simulink model "chap05"  (R2021a)
settings: Solver=FixedStepDiscrete  StartTime=0.0  StopTime=inf  FixedStep=0.001  RelTol=1e-3
undefined symbols (not defined in the file): DiscIntNeverNeededParam, Header, Pose, X, Y, Z
libraries: robotlib x31
(part 7 of 9)

== system chap05/Subsystem16/Subsystem6/Subsystem3 ==
  utx : Inport
  vx : Inport  Port=2
  vy : Inport  Port=3
  vz : Inport  Port=4
  uty : Inport  Port=5
  ux : Inport  Port=6
  uy : Inport  Port=7
  uz : Inport  Port=8
  utz : Inport  Port=9
  switch : Inport  Port=10
  Add3 : Sum  Inputs=-+
  Add4 : Sum  Inputs=-+
  Add5 : Sum  Inputs=-+
  Demux : Demux  Outputs=3
  Demux1 : Demux  Outputs=3
  Discrete-Time Integrator1 : DiscreteIntegrator  SampleTime=-1  ICPrevOutput=DiscIntNeverNeededParam  ICPrevScaledInput=DiscIntNeverNeededParam
  Discrete-Time Integrator2 : DiscreteIntegrator  SampleTime=-1  ICPrevOutput=DiscIntNeverNeededParam  ICPrevScaledInput=DiscIntNeverNeededParam
  Discrete-Time Integrator8 : DiscreteIntegrator  SampleTime=-1  ICPrevOutput=DiscIntNeverNeededParam  ICPrevScaledInput=DiscIntNeverNeededParam
  MATLAB Function : MATLAB Function  TreatAsAtomicUnit=on
  MATLAB Function1 : MATLAB Function  TreatAsAtomicUnit=on
  MATLAB Function2 : MATLAB Function  TreatAsAtomicUnit=on
  Mux : Mux  Inputs=3
  Mux1 : Mux  Inputs=3
  Subsystem : Subsystem
  Subsystem1 : Subsystem
  Subsystem2 : Subsystem
      settings: PortSchema="{\"entries\":[{\"content\":{\"sides\":[{\"content\":{\"connectorIds\":[\"In1\"]},\"type\":\"ConnectorPlacement.EquallySpacedRectSide\",\"uuid\":\"fc08b57d-5108-4bb3-894e-d1527c9ee9b9\"},{\"content\":{\"connectorIds\":[\"Out1\",\"Out2\",\"Out3\",\"Out4\"],\"side\":\"RIGHT\"},\"type\":\"ConnectorPlacement.EquallySpacedRectSide\",\"uuid\":\"5f28f464-9d6d-4ee7-848e-113b4b51ead6\"},{\"content\":{\"connectorIds\":[],\"side\":\"TOP\"},\"type\":\"ConnectorPlacement.EquallySpacedRectSide\",\"uuid\":\"5cca314e-822b-43eb-ac4d-78622e8ed582\"},{\"content\":{\"connectorIds\":[\"In2\"],\"side\":\"BOTTOM\"},\"type\":\"ConnectorPlacement.EquallySpacedRectSide\",\"uuid\":\"aa07b2d0-4f6e-4d8e-96de-14c35ee3da88\"}]},\"type\":\"ConnectorPlacement.EquallySpacedConnector\",\"uuid\":\"246d6f2c-2f9e-403c-b810-eff9b0fc0735\"}],\"packageUris\":[\"http://schema.mathworks.com/mf0/Connector/R2020b\"],\"version\":\"1.0\"}"
  Subsystem3 : Subsystem
  Subtract1 : Sum  Inputs=++++
  Subtract2 : Sum  Inputs=+-
  Subtract3 : Sum  Inputs=+-
  Subtract4 : Sum  Inputs=+-
  Switch1 : Switch  Criteria=u2 > Threshold  Threshold=1
  Switch2 : Switch  Criteria=u2 > Threshold  Threshold=1
  Switch3 : Switch  Criteria=u2 > Threshold  Threshold=1
  udtx : Outport
  udty : Outport  Port=2
  udtz : Outport  Port=3
  wires:
  Subsystem3/1(Out1) -> Subtract1/2
  Subsystem2/2(k2) -> Subsystem3/2(k2)
  Subsystem1/1(Out1) -> Subtract1/1
  Subsystem2/1(k1) -> Subsystem1/2(k1)
  Subtract4/1 -> MATLAB Function2/1(u)
  Subtract3/1 -> MATLAB Function1/1(u)
  Subtract2/1 -> MATLAB Function/1(u)
  Demux/3 -> Discrete-Time Integrator8/1
  Demux/1 -> Discrete-Time Integrator2/1
  Demux/2 -> Discrete-Time Integrator1/1
  Discrete-Time Integrator2/1 -> Subtract2/1
  Discrete-Time Integrator1/1 -> Subtract3/1
  Discrete-Time Integrator8/1 -> Subtract4/1
  Mux1/1 -> Subtract1/4
  ux/1 -> Mux1/1
  uy/1 -> Mux1/2
  uz/1 -> Mux1/3
  vx/1 -> Subtract2/2
  Subsystem2/4(k4) -> Subsystem/3(k4)
  Subsystem/1(z2) -> Demux1/1, Subtract1/3  "od6"
  Subsystem2/3(k3) -> Subsystem/2(k3)
  Subtract1/1 -> Demux/1
  Mux/1 -> Subsystem1/1(e1), Subsystem3/1(e1), Subsystem2/1(e1), Subsystem/1(e1)
  utx/1 -> Switch1/3, Add3/2
  uty/1 -> Switch2/3, Add5/2
  utz/1 -> Switch3/3, Add4/2
  vy/1 -> Subtract3/2
  vz/1 -> Subtract4/2
  MATLAB Function/1(y) -> Mux/1
  MATLAB Function1/1(y) -> Mux/2
  MATLAB Function2/1(y) -> Mux/3
  switch/1 -> [switch], Switch3/2, Switch1/2, Switch2/2
  [switch] -> Subsystem2/2(switch)
  Add3/1 -> Switch1/1
  Add5/1 -> Switch2/1
  Add4/1 -> Switch3/1
  Switch1/1 -> udtx/1
  Switch2/1 -> udty/1
  Switch3/1 -> udtz/1
  Demux1/1 -> Add3/1
  Demux1/2 -> Add5/1
  Demux1/3 -> Add4/1

== system chap05/Subsystem16/Subsystem6/Subsystem4 ==
  vx6 : Inport
  vx0 : Inport  Port=2
  utx : Inport  Port=3
  gain : Inport  Port=4
  switch : Inport  Port=5
  Add1 : Sum  Inputs=--+
  Constant1 : Constant  Value=0.08
  Constant2 : Constant  Value=10
  Product : Product
  Product1 : Product
  Product2 : Product
  Subsystem : Subsystem
  Subtract : Sum  Inputs=+--
  Switch1 : Switch  Criteria=u2 > Threshold  Threshold=1
  Tanh : Trigonometry  Operator=tanh
  ux : Outport
  Sx : Outport  Port=2
  wires:
  Add1/1 -> Switch1/1
  utx/1 -> [A], Subsystem/2(zt3)
  Subsystem/1(Out1) -> Subtract/3
  Product/1 -> Add1/2
  vx6/1 -> Subtract/1
  Product2/1 -> Tanh/1
  Tanh/1 -> Product/1
  gain/1 -> Product/2
  [A] -> Add1/3
  Constant2/1 -> Product2/2
  Product1/1 -> Add1/1
  Subtract/1 -> Sx/1, Product1/2, Product2/1
  vx0/1 -> Subtract/2
  switch/1 -> [switch], Subsystem/1(switch)
  [A] -> Switch1/3
  [switch] -> Switch1/2
  Switch1/1 -> ux/1
  Constant1/1 -> Product1/1

== system chap05/Subsystem16/Subsystem6/Subsystem5 ==
  vy6 : Inport
  vy0 : Inport  Port=2
  uty : Inport  Port=3
  gain : Inport  Port=4
  switch : Inport  Port=5
  Add1 : Sum  Inputs=--+
  Constant1 : Constant  Value=0.08
  Constant2 : Constant  Value=10
  Product : Product
  Product1 : Product
  Product2 : Product
  Subsystem : Subsystem
  Subtract : Sum  Inputs=+--
  Switch1 : Switch  Criteria=u2 > Threshold  Threshold=1
  Tanh : Trigonometry  Operator=tanh
  uy : Outport
  Sz : Outport  Port=2
  wires:
  Switch1/1 -> uy/1
  [switch] -> Switch1/2
  [A] -> Switch1/3
  switch/1 -> Subsystem/1(switch), [switch]
  vy0/1 -> Subtract/2
  Subtract/1 -> Product2/1, Product1/2, Sz/1
  Constant1/1 -> Product1/1
  Product1/1 -> Add1/1
  Constant2/1 -> Product2/2
  [A] -> Add1/3
  gain/1 -> Product/2
  Tanh/1 -> Product/1
  Product2/1 -> Tanh/1
  vy6/1 -> Subtract/1
  Product/1 -> Add1/2
  Subsystem/1(Out1) -> Subtract/3
  uty/1 -> Subsystem/2(zt3), [A]
  Add1/1 -> Switch1/1

== system chap05/Subsystem16/Subsystem6/Subsystem6 ==
  xx6 : Inport
  xx0 : Inport  Port=2
  xx1 : Inport  Port=3
  xx2 : Inport  Port=4
  vx6 : Inport  Port=5
  vx0 : Inport  Port=6
  vx1 : Inport  Port=7
  vx2 : Inport  Port=8
  Add : Sum
  Add1 : Sum  Inputs=-+
  Add10 : Sum  Inputs=-+
  Add2 : Sum  Inputs=+-
  Add4 : Sum  Inputs=-+
  Add5 : Sum  Inputs=+++
  Add6 : Sum  Inputs=+-
  Add8 : Sum  Inputs=+++
  Add9 : Sum  Inputs=+-
  Constant : Constant  Value=0.75
  Constant1 : Constant  Value=0.85
  Constant3 : Constant  Value=1.2
  Constant{4..5,7..8} (4 alike) : Constant  Value=1.5
  Constant6 : Constant  Value=1.2
  Gain : Gain  Gain=-1
  Product{1,3..9} (8 alike) : Product
  utx : Outport
  wires:
  Product9/1 -> Add8/2
  Product8/1 -> Add8/1
  Add9/1 -> Product9/1
  Constant6/1 -> Product9/2
  Add10/1 -> Product8/2
  Constant5/1 -> Product8/1
  Add8/1 -> Product1/2
  Product4/1 -> Add5/2
  Product5/1 -> Add5/3
  Constant4/1 -> Product4/1
  Add4/1 -> Product4/2
  xx6/1 -> Add1/2, Add2/1, Add4/2
  Constant3/1 -> Product5/2
  Product6/1 -> Add/1
  Constant/1 -> Product6/1
  Constant1/1 -> Product1/1
  Product1/1 -> Add/2
  Add2/1 -> Product5/1
  Add5/1 -> Product6/2
  xx2/1 -> Add4/1
  xx1/1 -> Add2/2
  vx1/1 -> Add9/2
  vx2/1 -> Add10/1
  vx6/1 -> Add6/1, Add9/1, Add10/2
  xx0/1 -> Add1/1
  Constant7/1 -> Product3/1
  Add1/1 -> Product3/2
  Product3/1 -> Add5/1
  vx0/1 -> Add6/2
  Constant8/1 -> Product7/2
  Add6/1 -> Product7/1
  Product7/1 -> Add8/3
  Gain/1 -> utx/1
  Add/1 -> Gain/1

== system chap05/Subsystem16/Subsystem6/Subsystem7 ==
  vz6 : Inport
  vz0 : Inport  Port=2
  utz : Inport  Port=3
  gain : Inport  Port=4
  switch : Inport  Port=5
  Add1 : Sum  Inputs=--+
  Constant1 : Constant  Value=0.08
  Constant2 : Constant  Value=10
  Product : Product
  Product1 : Product
  Product2 : Product
  Subsystem : Subsystem
  Subtract : Sum  Inputs=+--
  Switch1 : Switch  Criteria=u2 > Threshold  Threshold=1
  Tanh : Trigonometry  Operator=tanh
  uz : Outport
  Sz : Outport  Port=2
  wires:
  Add1/1 -> Switch1/1
  utz/1 -> [A], Subsystem/2(zt3)
  Subsystem/1(Out1) -> Subtract/3
  Product/1 -> Add1/2
  vz6/1 -> Subtract/1
  Product2/1 -> Tanh/1
  Tanh/1 -> Product/1
  gain/1 -> Product/2
  [A] -> Add1/3
  Constant2/1 -> Product2/2
  Product1/1 -> Add1/1
  Constant1/1 -> Product1/1
  Subtract/1 -> Sz/1, Product1/2, Product2/1
  vz0/1 -> Subtract/2
  switch/1 -> [switch], Subsystem/1(switch)
  [A] -> Switch1/3
  [switch] -> Switch1/2
  Switch1/1 -> uz/1

== system chap05/Subsystem16/Subsystem6/Subsystem8 ==
  Sx : Inport
  Sy : Inport  Port=2
  Sz : Inport  Port=3
  vx : Inport  Port=4
  vy : Inport  Port=5
  vz : Inport  Port=6
  switch : Inport  Port=7
  Constant{,1..3} (4 alike) : Constant  Value=0.1
  Discrete-Time Integrator1 : DiscreteIntegrator  gainval=1  InitialCondition=0.05  SampleTime=-1  ICPrevOutput=DiscIntNeverNeededParam  ICPrevScaledInput=DiscIntNeverNeededParam
  Discrete-Time Integrator2 : DiscreteIntegrator  gainval=1  InitialCondition=0.025  SampleTime=-1  ICPrevOutput=DiscIntNeverNeededParam  ICPrevScaledInput=DiscIntNeverNeededParam
  Discrete-Time Integrator3 : DiscreteIntegrator  gainval=1  InitialCondition=0.01  SampleTime=-1  ICPrevOutput=DiscIntNeverNeededParam  ICPrevScaledInput=DiscIntNeverNeededParam
  MATLAB Function : MATLAB Function  TreatAsAtomicUnit=on
  MATLAB Function1 : MATLAB Function  TreatAsAtomicUnit=on
  Mux1 : Mux  Inputs=3
  Mux3 : Mux  Inputs=3
  Product{1..4,6..8} (7 alike) : Product
  Square : Math  Operator=square  SaturateOnIntegerOverflow=on
  Square1 : Math  Operator=square  SaturateOnIntegerOverflow=on
  Subsystem : Subsystem
      settings: PortSchema="{\"entries\":[{\"content\":{\"sides\":[{\"content\":{\"connectorIds\":[\"In1\"]},\"type\":\"ConnectorPlacement.EquallySpacedRectSide\",\"uuid\":\"50b1559e-7173-4ba8-93e6-314f6d9df527\"},{\"content\":{\"connectorIds\":[\"Out1\"],\"side\":\"RIGHT\"},\"type\":\"ConnectorPlacement.EquallySpacedRectSide\",\"uuid\":\"be527bac-0bcc-4faf-a185-0382edae0189\"},{\"content\":{\"connectorIds\":[\"In2\"],\"side\":\"TOP\"},\"type\":\"ConnectorPlacement.EquallySpacedRectSide\",\"uuid\":\"4c8ef68d-7cf5-4d15-9758-89dbc1169805\"}]},\"type\":\"ConnectorPlacement.EquallySpacedConnector\",\"uuid\":\"3c2ee67b-c3c9-431a-8107-6d5cd22b236e\"}],\"packageUris\":[\"http://schema.mathworks.com/mf0/Connector/R2020b\"],\"version\":\"1.0\"}"
  Subsystem1 : Subsystem
      settings: PortSchema="{\"entries\":[{\"content\":{\"sides\":[{\"content\":{\"connectorIds\":[\"In1\"]},\"type\":\"ConnectorPlacement.EquallySpacedRectSide\",\"uuid\":\"50b1559e-7173-4ba8-93e6-314f6d9df527\"},{\"content\":{\"connectorIds\":[\"Out1\"],\"side\":\"RIGHT\"},\"type\":\"ConnectorPlacement.EquallySpacedRectSide\",\"uuid\":\"be527bac-0bcc-4faf-a185-0382edae0189\"},{\"content\":{\"connectorIds\":[\"In2\"],\"side\":\"TOP\"},\"type\":\"ConnectorPlacement.EquallySpacedRectSide\",\"uuid\":\"4c8ef68d-7cf5-4d15-9758-89dbc1169805\"}]},\"type\":\"ConnectorPlacement.EquallySpacedConnector\",\"uuid\":\"3c2ee67b-c3c9-431a-8107-6d5cd22b236e\"}],\"packageUris\":[\"http://schema.mathworks.com/mf0/Connector/R2020b\"],\"version\":\"1.0\"}"
  Subsystem2 : Subsystem
      settings: PortSchema="{\"entries\":[{\"content\":{\"sides\":[{\"content\":{\"connectorIds\":[\"In1\"]},\"type\":\"ConnectorPlacement.EquallySpacedRectSide\",\"uuid\":\"50b1559e-7173-4ba8-93e6-314f6d9df527\"},{\"content\":{\"connectorIds\":[\"Out1\"],\"side\":\"RIGHT\"},\"type\":\"ConnectorPlacement.EquallySpacedRectSide\",\"uuid\":\"be527bac-0bcc-4faf-a185-0382edae0189\"},{\"content\":{\"connectorIds\":[\"In2\"],\"side\":\"TOP\"},\"type\":\"ConnectorPlacement.EquallySpacedRectSide\",\"uuid\":\"4c8ef68d-7cf5-4d15-9758-89dbc1169805\"}]},\"type\":\"ConnectorPlacement.EquallySpacedConnector\",\"uuid\":\"3c2ee67b-c3c9-431a-8107-6d5cd22b236e\"}],\"packageUris\":[\"http://schema.mathworks.com/mf0/Connector/R2020b\"],\"version\":\"1.0\"}"
  Subtract1 : Sum  Inputs=++++
  Subtract2 : Sum  Inputs=+-
  Subtract3 : Sum  Inputs=+-
  Subtract4 : Sum  Inputs=+-
  " gain" : Outport
  wires:
  [switch] -> Subsystem2/2(switch)
  [switch] -> Subsystem1/2(switch)
  [switch] -> Subsystem/2(switch)
  switch/1 -> [switch]
  Subsystem1/1(Out1) -> Discrete-Time Integrator2/1
  Subsystem2/1(Out1) -> Discrete-Time Integrator3/1
  Subsystem/1(Out1) -> Discrete-Time Integrator1/1
  [norm_V] -> Product8/2
  Square1/1 -> Product4/1
  [norm_V] -> Square1/1
  [norm_V] -> Product1/1
  [norm_V] -> Square/1
  [norm_S] -> Product3/1
  [norm_S] -> Product8/1
  [norm_S] -> Subtract2/1
  MATLAB Function/1(y) -> [norm_S]
  vy/1 -> Mux1/2
  vz/1 -> Mux1/3
  vx/1 -> Mux1/1
  Sz/1 -> Mux3/3
  Sy/1 -> Mux3/2
  Sx/1 -> Mux3/1
  Constant3/1 -> Product7/1
  Constant2/1 -> Product6/1
  Constant1/1 -> Subtract1/4
  Product4/1 -> Subtract1/3
  MATLAB Function1/1(y) -> [norm_V]
  Constant/1 -> Product2/1
  Mux1/1 -> MATLAB Function1/1(u)
  Square/1 -> Product3/2
  Mux3/1 -> MATLAB Function/1(u)
  Discrete-Time Integrator3/1 -> Product2/2, Product4/2  "K2"
  Product2/1 -> Subtract4/2
  Product3/1 -> Subtract4/1
  Subtract4/1 -> Subsystem2/1(In1)
  Subtract3/1 -> Subsystem1/1(In1)
  Product8/1 -> Subtract3/1
  Product7/1 -> Subtract3/2
  Discrete-Time Integrator2/1 -> Product1/2, Product7/2  "K1"
  Product6/1 -> Subtract2/2
  Discrete-Time Integrator1/1 -> Subtract1/1, Product6/2  "K0"
  Subtract2/1 -> Subsystem/1(In1)
  Product1/1 -> Subtract1/2
  Subtract1/1 -> " gain"/1

== system chap05/Subsystem16/Subsystem8/L+B ==
  Add : Sum
  Constant1 : Constant  Value=|
      | [2.5 0 0 0 0 0
      |      0 2.8 0 0 0 0
      |      0 0 2.8 0 0 0
      |      0 0 0 2.5 0 0
      |      0 0 0 0 2.7 0
      |      0 0 0 0 0 2.7]
  Constant2 : Constant  Value=|
      | [0.0 0.8 0.5 0.0 0.0 1.2
      |      0.8 0.0 0.0 0.5 0.0 1.5
      |      0.5 0.0 0.0 0.8 1.5 0.0
      |      0.0 0.5 0.8 0.0 1.2 0.0
      |      0.0 0.0 1.5 1.2 0.0 0.0
      |      1.2 1.5 0.0 0.0 0.0 0.0]
  Constant3 : Constant  Value=|
      | [0.0 0.0 0.0 0.0 0.0 0.0
      |      0.0 0.0 0.0 0.0 0.0 0.0
      |      0.0 0.0 0.0 0.0 0.0 0.0
      |      0.0 0.0 0.0 0.0 0.0 0.0
      |      0.0 0.0 0.0 0.0 1.5 0.0
      |      0.0 0.0 0.0 0.0 0.0 1.5]
  Subtract : Sum  Inputs=+-
  u : Outport
  wires:
  Constant2/1 -> Subtract/2
  Constant1/1 -> Subtract/1
  Subtract/1 -> Add/1
  Add/1 -> u/1
  Constant3/1 -> Add/2

== system chap05/Subsystem16/Subsystem8/Subsystem1 ==
  xy4 : Inport
  xy2 : Inport  Port=2
  xy3 : Inport  Port=3
  xy5 : Inport  Port=4
  vy4 : Inport  Port=5
  vy2 : Inport  Port=6
  vy3 : Inport  Port=7
  vy5 : Inport  Port=8
  Add : Sum
  Add{1,4,6,8} (4 alike) : Sum  Inputs=-+
  Add2 : Sum  Inputs=+-
  Add5 : Sum  Inputs=+++
  Add7 : Sum  Inputs=+-
  Add9 : Sum  Inputs=+++
  Constant : Constant  Value=0.75
  Constant1 : Constant  Value=0.85
  Constant2 : Constant  Value=0.8
  Constant3 : Constant  Value=0.8
  Constant4 : Constant  Value=0.5
  Constant5 : Constant  Value=1.2
  Constant6 : Constant  Value=0.5
  Constant7 : Constant  Value=1.2
  Product{1,3..9} (8 alike) : Product
  p4y : Outport
  wires:
  Product8/1 -> Add9/2
  Product9/1 -> Add9/3
  Constant2/1 -> Product8/1
  Add8/1 -> Product8/2
  vy4/1 -> Add6/2, Add8/2, Add7/1
  Constant6/1 -> Product9/2
  Add7/1 -> Product9/1
  vy3/1 -> Add8/1
  vy2/1 -> Add7/2
  vy5/1 -> Add6/1
  Constant7/1 -> Product7/1
  Add6/1 -> Product7/2
  Product7/1 -> Add9/1
  Product3/1 -> Add5/1
  Add1/1 -> Product3/2
  Constant5/1 -> Product3/1
  xy5/1 -> Add1/1
  xy2/1 -> Add2/2
  xy3/1 -> Add4/1
  Add/1 -> p4y/1
  Add5/1 -> Product6/2
  Add2/1 -> Product5/1
  Product1/1 -> Add/2
  Constant1/1 -> Product1/1
  Constant/1 -> Product6/1
  Product6/1 -> Add/1
  Constant4/1 -> Product5/2
  xy4/1 -> Add2/1, Add4/2, Add1/2
  Add4/1 -> Product4/2
  Constant3/1 -> Product4/1
  Product5/1 -> Add5/3
  Product4/1 -> Add5/2
  Add9/1 -> Product1/2

== system chap05/Subsystem16/Subsystem8/Subsystem2 ==
  xz4 : Inport
  xx2 : Inport  Port=2
  xz3 : Inport  Port=3
  xz5 : Inport  Port=4
  vz4 : Inport  Port=5
  vz2 : Inport  Port=6
  vz3 : Inport  Port=7
  vz5 : Inport  Port=8
  Add : Sum
  Add{1,4,6,8} (4 alike) : Sum  Inputs=-+
  Add2 : Sum  Inputs=+-
  Add5 : Sum  Inputs=+++
  Add7 : Sum  Inputs=+-
  Add9 : Sum  Inputs=+++
  Constant : Constant  Value=0.75
  Constant1 : Constant  Value=0.85
  Constant2 : Constant  Value=0.8
  Constant3 : Constant  Value=0.8
  Constant4 : Constant  Value=0.5
  Constant5 : Constant  Value=1.2
  Constant6 : Constant  Value=0.5
  Constant7 : Constant  Value=1.2
  Product{1,3..9} (8 alike) : Product
  p4z : Outport
  wires:
  Add9/1 -> Product1/2
  Product4/1 -> Add5/2
  Product5/1 -> Add5/3
  Constant3/1 -> Product4/1
  Add4/1 -> Product4/2
  xz4/1 -> Add1/2, Add4/2, Add2/1
  Constant4/1 -> Product5/2
  Product6/1 -> Add/1
  Constant/1 -> Product6/1
  Constant1/1 -> Product1/1
  Product1/1 -> Add/2
  Add2/1 -> Product5/1
  Add5/1 -> Product6/2
  Add/1 -> p4z/1
  xz3/1 -> Add4/1
  xx2/1 -> Add2/2
  xz5/1 -> Add1/1
  Constant5/1 -> Product3/1
  Add1/1 -> Product3/2
  Product3/1 -> Add5/1
  Product7/1 -> Add9/1
  Add6/1 -> Product7/2
  Constant7/1 -> Product7/1
  vz5/1 -> Add6/1
  vz2/1 -> Add7/2
  vz3/1 -> Add8/1
  Add7/1 -> Product9/1
  Constant6/1 -> Product9/2
  vz4/1 -> Add7/1, Add8/2, Add6/2
  Add8/1 -> Product8/2
  Constant2/1 -> Product8/1
  Product9/1 -> Add9/3
  Product8/1 -> Add9/2

== system chap05/Subsystem16/Subsystem8/Subsystem3 ==
  xyk : Inport
  xy : Inport  Port=2
  vyk : Inport  Port=3
  vy : Inport  Port=4
  Add : Sum
  Add4 : Sum  Inputs=-+
  Add8 : Sum  Inputs=-+
  Constant : Constant  Value=0.75
  Constant1 : Constant  Value=0.85
  Product1 : Product
  Product6 : Product
  ey : Outport
  wires:
  vyk/1 -> Add8/2
  vy/1 -> Add8/1
  xy/1 -> Add4/1
  Add/1 -> ey/1
  Add4/1 -> Product6/2
  Product1/1 -> Add/2
  Constant1/1 -> Product1/1
  Constant/1 -> Product6/1
  Product6/1 -> Add/1
  xyk/1 -> Add4/2
  Add8/1 -> Product1/2

== system chap05/Subsystem16/Subsystem8/Subsystem4 ==
  xzk : Inport
  xz : Inport  Port=2
  vzk : Inport  Port=3
  vz : Inport  Port=4
  Add : Sum
  Add4 : Sum  Inputs=-+
  Add8 : Sum  Inputs=-+
  Constant : Constant  Value=0.75
  Constant1 : Constant  Value=0.85
  Product1 : Product
  Product6 : Product
  ez : Outport
  wires:
  Add8/1 -> Product1/2
  xzk/1 -> Add4/2
  Product6/1 -> Add/1
  Constant/1 -> Product6/1
  Constant1/1 -> Product1/1
  Product1/1 -> Add/2
  Add4/1 -> Product6/2
  Add/1 -> ez/1
  xz/1 -> Add4/1
  vz/1 -> Add8/1
  vzk/1 -> Add8/2

== system chap05/Subsystem16/Subsystem8/Subsystem5 ==
  xxk : Inport
  xx : Inport  Port=2
  vxk : Inport  Port=3
  vx : Inport  Port=4
  Add : Sum
  Add4 : Sum  Inputs=-+
  Add8 : Sum  Inputs=-+
  Constant : Constant  Value=0.75
  Constant1 : Constant  Value=0.85
  Product1 : Product
  Product6 : Product
  ex : Outport
  wires:
  Add8/1 -> Product1/2
  xxk/1 -> Add4/2
  Product6/1 -> Add/1
  Constant/1 -> Product6/1
  Constant1/1 -> Product1/1
  Product1/1 -> Add/2
  Add4/1 -> Product6/2
  Add/1 -> ex/1
  xx/1 -> Add4/1
  vx/1 -> Add8/1
  vxk/1 -> Add8/2

== system chap05/Subsystem16/Subsystem8/Subsystem6 ==
  xx4 : Inport
  xx2 : Inport  Port=2
  xx3 : Inport  Port=3
  xx5 : Inport  Port=4
  vx4 : Inport  Port=5
  vx2 : Inport  Port=6
  vx3 : Inport  Port=7
  vx5 : Inport  Port=8
  Add : Sum
  Add{1,4,6,8} (4 alike) : Sum  Inputs=-+
  Add2 : Sum  Inputs=+-
  Add5 : Sum  Inputs=+++
  Add7 : Sum  Inputs=+-
  Add9 : Sum  Inputs=+++
  Constant : Constant  Value=0.75
  Constant1 : Constant  Value=0.85
  Constant2 : Constant  Value=0.8
  Constant3 : Constant  Value=0.8
  Constant4 : Constant  Value=0.5
  Constant5 : Constant  Value=1.2
  Constant6 : Constant  Value=0.5
  Constant7 : Constant  Value=1.2
  Product{1,3..9} (8 alike) : Product
  p4x : Outport
  wires:
  Add9/1 -> Product1/2
  Product4/1 -> Add5/2
  Product5/1 -> Add5/3
  Constant3/1 -> Product4/1
  Add4/1 -> Product4/2
  xx4/1 -> Add1/2, Add4/2, Add2/1
  Constant4/1 -> Product5/2
  Product6/1 -> Add/1
  Constant/1 -> Product6/1
  Constant1/1 -> Product1/1
  Product1/1 -> Add/2
  Add2/1 -> Product5/1
  Add5/1 -> Product6/2
  Add/1 -> p4x/1
  xx3/1 -> Add4/1
  xx2/1 -> Add2/2
  xx5/1 -> Add1/1
  Constant5/1 -> Product3/1
  Add1/1 -> Product3/2
  Product3/1 -> Add5/1
  Product7/1 -> Add9/1
  Add6/1 -> Product7/2
  Constant7/1 -> Product7/1
  vx5/1 -> Add6/1
  vx2/1 -> Add7/2
  vx3/1 -> Add8/1
  Add7/1 -> Product9/1
  Constant6/1 -> Product9/2
  vx4/1 -> Add7/1, Add8/2, Add6/2
  Add8/1 -> Product8/2
  Constant2/1 -> Product8/1
  Product9/1 -> Add9/3
  Product8/1 -> Add9/2

== system chap05/Subsystem16/Subsystem/Subsystem11/Subsystem ==
  switch : Inport
  zt3 : Inport  Port=2
  Constant4 : Constant  Value=0
  Discrete-Time Integrator : DiscreteIntegrator  SampleTime=-1  UpperSaturationLimit=100  LowerSaturationLimit=-100  ICPrevOutput=DiscIntNeverNeededParam  ICPrevScaledInput=DiscIntNeverNeededParam
  Logical Operator : Logic  AllPortsSameDT=off  OutDataTypeStr=boolean
  MATLAB Function : MATLAB Function  TreatAsAtomicUnit=on
  Relational Operator : RelationalOperator  Operator===  OutDataTypeStr=boolean  RndMeth=Simplest
  Saturation1 : Saturate  UpperLimit=0.25  LowerLimit=-0.25
  Sign : Signum
  Sign1 : Signum
  Subsystem : Subsystem
      settings: PortSchema="{\"entries\":[{\"content\":{\"sides\":[{\"content\":{\"connectorIds\":[\"In1\"]},\"type\":\"ConnectorPlacement.EquallySpacedRectSide\",\"uuid\":\"50b1559e-7173-4ba8-93e6-314f6d9df527\"},{\"content\":{\"connectorIds\":[\"Out1\"],\"side\":\"RIGHT\"},\"type\":\"ConnectorPlacement.EquallySpacedRectSide\",\"uuid\":\"be527bac-0bcc-4faf-a185-0382edae0189\"},{\"content\":{\"connectorIds\":[\"In2\"],\"side\":\"TOP\"},\"type\":\"ConnectorPlacement.EquallySpacedRectSide\",\"uuid\":\"4c8ef68d-7cf5-4d15-9758-89dbc1169805\"}]},\"type\":\"ConnectorPlacement.EquallySpacedConnector\",\"uuid\":\"3c2ee67b-c3c9-431a-8107-6d5cd22b236e\"}],\"packageUris\":[\"http://schema.mathworks.com/mf0/Connector/R2020b\"],\"version\":\"1.0\"}"
  Switch : Switch  Criteria=u2 > Threshold
  Out1 : Outport
  wires:
  MATLAB Function/1(y) -> Logical Operator/1
  Relational Operator/1 -> Logical Operator/2
  Constant4/1 -> Switch/1
  Sign1/1 -> Relational Operator/1
  Subsystem/1(Out1) -> Sign1/1, Switch/3
  Saturation1/1 -> Out1/1, MATLAB Function/2(u2)
  Discrete-Time Integrator/1 -> Saturation1/1, MATLAB Function/1(u1), Sign/1
  Sign/1 -> Relational Operator/2
  Logical Operator/1 -> Switch/2
  Switch/1 -> Discrete-Time Integrator/1
  zt3/1 -> Subsystem/1(zt3)
  switch/1 -> Subsystem/2(switch)

== system chap05/Subsystem16/Subsystem/Subsystem3/Subsystem ==
  e1 : Inport
  k3 : Inport  Port=2
  k4 : Inport  Port=3
  Add : Sum
  Constant3 : Constant  Value=-1
  Constant4 : Constant  Value=-1
  Discrete-Time Integrator1 : DiscreteIntegrator  SampleTime=-1  ICPrevOutput=DiscIntNeverNeededParam  ICPrevScaledInput=DiscIntNeverNeededParam
  Divide : Product  Inputs=*/
  MATLAB Function : MATLAB Function  TreatAsAtomicUnit=on
  Product3 : Product  Inputs=3
  Product5 : Product  Inputs=3
  z2 : Outport
  wires:
  Constant4/1 -> Product5/1
  Product5/1 -> Add/2
  Discrete-Time Integrator1/1 -> z2/1
  k3/1 -> Product3/3
  k4/1 -> Product5/3
  Divide/1 -> Add/1
  Add/1 -> Discrete-Time Integrator1/1
  Constant3/1 -> Product3/1
  e1/1 -> Product5/2, MATLAB Function/1(u), Product3/2
  MATLAB Function/1(y) -> Divide/2
  Product3/1 -> Divide/1

== system chap05/Subsystem16/Subsystem/Subsystem3/Subsystem1 ==
  e1 : Inport
  k1 : Inport  Port=2
  Constant : Constant  Value=-1
  Divide : Product  Inputs=*/
  MATLAB Function : MATLAB Function  TreatAsAtomicUnit=on
  Product : Product  Inputs=3
  Out1 : Outport
  wires:
  e1/1 -> Product/2, MATLAB Function/1(u)
  Divide/1 -> Out1/1
  Constant/1 -> Product/1
  k1/1 -> Product/3
  MATLAB Function/1(y) -> Divide/2
  Product/1 -> Divide/1

== system chap05/Subsystem16/Subsystem/Subsystem3/Subsystem2 ==
  e1 : Inport
  switch : Inport  Port=2
  Constant1 : Constant  Value=0.1
  MATLAB Function : MATLAB Function  TreatAsAtomicUnit=on
  Product{,1..3,6} (5 alike) : Product
  Sqrt : Sqrt  SaturateOnIntegerOverflow=on
  Square : Math  Operator=square  SaturateOnIntegerOverflow=on
  Subsystem : Subsystem
      settings: PortSchema="{\"entries\":[{\"content\":{\"sides\":[{\"content\":{\"connectorIds\":[\"In1\"]},\"type\":\"ConnectorPlacement.EquallySpacedRectSide\",\"uuid\":\"12a3f2f0-a297-420d-b26a-5f62088d5514\"},{\"content\":{\"connectorIds\":[\"Out1\"],\"side\":\"RIGHT\"},\"type\":\"ConnectorPlacement.EquallySpacedRectSide\",\"uuid\":\"62e35448-e0a3-4495-a6db-77deef7aa7b4\"},{\"content\":{\"connectorIds\":[\"In2\"],\"side\":\"TOP\"},\"type\":\"ConnectorPlacement.EquallySpacedRectSide\",\"uuid\":\"3e6c604a-b26b-4ac2-9bdc-2cdec7247e53\"}]},\"type\":\"ConnectorPlacement.EquallySpacedConnector\",\"uuid\":\"6331fe4a-63c7-4003-9b0d-be968a8635fa\"}],\"packageUris\":[\"http://schema.mathworks.com/mf0/Connector/R2020b\"],\"version\":\"1.0\"}"
  Subtract2 : Sum  Inputs=+-
  c1 : Constant  Value=0.1
  c2 : Constant  Value=0.1
  c3 : Constant  Value=0.3
  c4 : Constant  Value=0.3
  k1 : Outport
  k2 : Outport  Port=2
  k3 : Outport  Port=3
  k4 : Outport  Port=4
  wires:
  c2/1 -> Product/2
  Product/1 -> k2/1
  c3/1 -> Product1/1
  Product1/1 -> k3/1
  c4/1 -> Product2/1
  Product2/1 -> k4/1
  c1/1 -> Product3/2
  Product3/1 -> k1/1
  Sqrt/1 -> Product3/1
  Square/1 -> Product2/2
  e1/1 -> MATLAB Function/1(u)
  Product6/1 -> Subtract2/2
  MATLAB Function/1(y) -> Subtract2/1
  Subtract2/1 -> Subsystem/1(In1)
  Constant1/1 -> Product6/1
  switch/1 -> Subsystem/2(switch)
  Subsystem/1(Out1) -> Product6/2, Sqrt/1, Product1/2, Square/1, Product/1

== system chap05/Subsystem16/Subsystem/Subsystem3/Subsystem3 ==
  e1 : Inport
  k2 : Inport  Port=2
  Constant2 : Constant  Value=-1
  Product2 : Product  Inputs=3
  Out1 : Outport
  wires:
  Product2/1 -> Out1/1
  e1/1 -> Product2/2
  k2/1 -> Product2/3
  Constant2/1 -> Product2/1

== system chap05/Subsystem16/Subsystem/Subsystem4/Subsystem ==
  switch : Inport
  zt3 : Inport  Port=2
  Constant4 : Constant  Value=0
  Discrete-Time Integrator : DiscreteIntegrator  SampleTime=-1  UpperSaturationLimit=100  LowerSaturationLimit=-100  ICPrevOutput=DiscIntNeverNeededParam  ICPrevScaledInput=DiscIntNeverNeededParam
  Logical Operator : Logic  AllPortsSameDT=off  OutDataTypeStr=boolean
  MATLAB Function : MATLAB Function  TreatAsAtomicUnit=on
  Relational Operator : RelationalOperator  Operator===  OutDataTypeStr=boolean  RndMeth=Simplest
  Saturation1 : Saturate  UpperLimit=0.25  LowerLimit=-0.25
  Sign : Signum
  Sign1 : Signum
  Subsystem : Subsystem
      settings: PortSchema="{\"entries\":[{\"content\":{\"sides\":[{\"content\":{\"connectorIds\":[\"In1\"]},\"type\":\"ConnectorPlacement.EquallySpacedRectSide\",\"uuid\":\"50b1559e-7173-4ba8-93e6-314f6d9df527\"},{\"content\":{\"connectorIds\":[\"Out1\"],\"side\":\"RIGHT\"},\"type\":\"ConnectorPlacement.EquallySpacedRectSide\",\"uuid\":\"be527bac-0bcc-4faf-a185-0382edae0189\"},{\"content\":{\"connectorIds\":[\"In2\"],\"side\":\"TOP\"},\"type\":\"ConnectorPlacement.EquallySpacedRectSide\",\"uuid\":\"4c8ef68d-7cf5-4d15-9758-89dbc1169805\"}]},\"type\":\"ConnectorPlacement.EquallySpacedConnector\",\"uuid\":\"3c2ee67b-c3c9-431a-8107-6d5cd22b236e\"}],\"packageUris\":[\"http://schema.mathworks.com/mf0/Connector/R2020b\"],\"version\":\"1.0\"}"
  Switch : Switch  Criteria=u2 > Threshold
  Out1 : Outport
  wires:
  MATLAB Function/1(y) -> Logical Operator/1
  Relational Operator/1 -> Logical Operator/2
  Constant4/1 -> Switch/1
  Sign1/1 -> Relational Operator/1
  Subsystem/1(Out1) -> Sign1/1, Switch/3
  Saturation1/1 -> Out1/1, MATLAB Function/2(u2)
  Discrete-Time Integrator/1 -> Saturation1/1, MATLAB Function/1(u1), Sign/1
  Sign/1 -> Relational Operator/2
  Logical Operator/1 -> Switch/2
  Switch/1 -> Discrete-Time Integrator/1
  zt3/1 -> Subsystem/1(zt3)
  switch/1 -> Subsystem/2(switch)

== system chap05/Subsystem16/Subsystem/Subsystem8/Subsystem ==
  In1 : Inport
  switch : Inport  Port=2
  Constant4 : Constant  Value=0
  Switch1 : Switch  Criteria=u2 > Threshold
  Out1 : Outport
  wires:
  In1/1 -> Switch1/1
  Switch1/1 -> Out1/1
  switch/1 -> Switch1/2
  Constant4/1 -> Switch1/3

== system chap05/Subsystem16/Subsystem/Subsystem8/Subsystem1 ==
  In1 : Inport
  switch : Inport  Port=2
  Constant4 : Constant  Value=0
  Switch1 : Switch  Criteria=u2 > Threshold
  Out1 : Outport
  wires:
  Constant4/1 -> Switch1/3
  switch/1 -> Switch1/2
  Switch1/1 -> Out1/1
  In1/1 -> Switch1/1

== system chap05/Subsystem16/Subsystem/Subsystem8/Subsystem2 ==
  In1 : Inport
  switch : Inport  Port=2
  Constant4 : Constant  Value=0
  Switch1 : Switch  Criteria=u2 > Threshold
  Out1 : Outport
  wires:
  In1/1 -> Switch1/1
  Switch1/1 -> Out1/1
  switch/1 -> Switch1/2
  Constant4/1 -> Switch1/3

== system chap05/Subsystem16/Subsystem/Subsystem9/Subsystem ==
  switch : Inport
  zt3 : Inport  Port=2
  Constant4 : Constant  Value=0
  Discrete-Time Integrator : DiscreteIntegrator  SampleTime=-1  UpperSaturationLimit=100  LowerSaturationLimit=-100  ICPrevOutput=DiscIntNeverNeededParam  ICPrevScaledInput=DiscIntNeverNeededParam
  Logical Operator : Logic  AllPortsSameDT=off  OutDataTypeStr=boolean
  MATLAB Function : MATLAB Function  TreatAsAtomicUnit=on
  Relational Operator : RelationalOperator  Operator===  OutDataTypeStr=boolean  RndMeth=Simplest
  Saturation1 : Saturate  UpperLimit=0.25  LowerLimit=-0.25
  Sign : Signum
  Sign1 : Signum
  Subsystem : Subsystem
      settings: PortSchema="{\"entries\":[{\"content\":{\"sides\":[{\"content\":{\"connectorIds\":[\"In1\"]},\"type\":\"ConnectorPlacement.EquallySpacedRectSide\",\"uuid\":\"50b1559e-7173-4ba8-93e6-314f6d9df527\"},{\"content\":{\"connectorIds\":[\"Out1\"],\"side\":\"RIGHT\"},\"type\":\"ConnectorPlacement.EquallySpacedRectSide\",\"uuid\":\"be527bac-0bcc-4faf-a185-0382edae0189\"},{\"content\":{\"connectorIds\":[\"In2\"],\"side\":\"TOP\"},\"type\":\"ConnectorPlacement.EquallySpacedRectSide\",\"uuid\":\"4c8ef68d-7cf5-4d15-9758-89dbc1169805\"}]},\"type\":\"ConnectorPlacement.EquallySpacedConnector\",\"uuid\":\"3c2ee67b-c3c9-431a-8107-6d5cd22b236e\"}],\"packageUris\":[\"http://schema.mathworks.com/mf0/Connector/R2020b\"],\"version\":\"1.0\"}"
  Switch : Switch  Criteria=u2 > Threshold
  Out1 : Outport
  wires:
  zt3/1 -> Subsystem/1(zt3)
  switch/1 -> Subsystem/2(switch)
  Switch/1 -> Discrete-Time Integrator/1
  Logical Operator/1 -> Switch/2
  Sign/1 -> Relational Operator/2
  Discrete-Time Integrator/1 -> Saturation1/1, Sign/1, MATLAB Function/1(u1)
  Saturation1/1 -> MATLAB Function/2(u2), Out1/1
  Subsystem/1(Out1) -> Switch/3, Sign1/1
  Sign1/1 -> Relational Operator/1
  Constant4/1 -> Switch/1
  Relational Operator/1 -> Logical Operator/2
  MATLAB Function/1(y) -> Logical Operator/1

== system chap05/Subsystem16/Subsystem1/Subsystem11/Subsystem ==
  switch : Inport
  zt3 : Inport  Port=2
  Constant4 : Constant  Value=0
  Discrete-Time Integrator : DiscreteIntegrator  SampleTime=-1  UpperSaturationLimit=100  LowerSaturationLimit=-100  ICPrevOutput=DiscIntNeverNeededParam  ICPrevScaledInput=DiscIntNeverNeededParam
  Logical Operator : Logic  AllPortsSameDT=off  OutDataTypeStr=boolean
  MATLAB Function : MATLAB Function  TreatAsAtomicUnit=on
  Relational Operator : RelationalOperator  Operator===  OutDataTypeStr=boolean  RndMeth=Simplest
  Saturation1 : Saturate  UpperLimit=0.25  LowerLimit=-0.25
  Sign : Signum
  Sign1 : Signum
  Subsystem : Subsystem
      settings: PortSchema="{\"entries\":[{\"content\":{\"sides\":[{\"content\":{\"connectorIds\":[\"In1\"]},\"type\":\"ConnectorPlacement.EquallySpacedRectSide\",\"uuid\":\"50b1559e-7173-4ba8-93e6-314f6d9df527\"},{\"content\":{\"connectorIds\":[\"Out1\"],\"side\":\"RIGHT\"},\"type\":\"ConnectorPlacement.EquallySpacedRectSide\",\"uuid\":\"be527bac-0bcc-4faf-a185-0382edae0189\"},{\"content\":{\"connectorIds\":[\"In2\"],\"side\":\"TOP\"},\"type\":\"ConnectorPlacement.EquallySpacedRectSide\",\"uuid\":\"4c8ef68d-7cf5-4d15-9758-89dbc1169805\"}]},\"type\":\"ConnectorPlacement.EquallySpacedConnector\",\"uuid\":\"3c2ee67b-c3c9-431a-8107-6d5cd22b236e\"}],\"packageUris\":[\"http://schema.mathworks.com/mf0/Connector/R2020b\"],\"version\":\"1.0\"}"
  Switch : Switch  Criteria=u2 > Threshold
  Out1 : Outport
  wires:
  MATLAB Function/1(y) -> Logical Operator/1
  Relational Operator/1 -> Logical Operator/2
  Constant4/1 -> Switch/1
  Sign1/1 -> Relational Operator/1
  Subsystem/1(Out1) -> Sign1/1, Switch/3
  Saturation1/1 -> Out1/1, MATLAB Function/2(u2)
  Discrete-Time Integrator/1 -> Saturation1/1, MATLAB Function/1(u1), Sign/1
  Sign/1 -> Relational Operator/2
  Logical Operator/1 -> Switch/2
  Switch/1 -> Discrete-Time Integrator/1
  zt3/1 -> Subsystem/1(zt3)
  switch/1 -> Subsystem/2(switch)

== system chap05/Subsystem16/Subsystem1/Subsystem3/Subsystem ==
  e1 : Inport
  k3 : Inport  Port=2
  k4 : Inport  Port=3
  Add : Sum
  Constant3 : Constant  Value=-1
  Constant4 : Constant  Value=-1
  Discrete-Time Integrator1 : DiscreteIntegrator  SampleTime=-1  ICPrevOutput=DiscIntNeverNeededParam  ICPrevScaledInput=DiscIntNeverNeededParam
  Divide : Product  Inputs=*/
  MATLAB Function : MATLAB Function  TreatAsAtomicUnit=on
  Product3 : Product  Inputs=3
  Product5 : Product  Inputs=3
  z2 : Outport
  wires:
  Constant4/1 -> Product5/1
  Product5/1 -> Add/2
  Discrete-Time Integrator1/1 -> z2/1
  k3/1 -> Product3/3
  k4/1 -> Product5/3
  Divide/1 -> Add/1
  Add/1 -> Discrete-Time Integrator1/1
  Constant3/1 -> Product3/1
  e1/1 -> Product5/2, MATLAB Function/1(u), Product3/2
  MATLAB Function/1(y) -> Divide/2
  Product3/1 -> Divide/1

== system chap05/Subsystem16/Subsystem1/Subsystem3/Subsystem1 ==
  e1 : Inport
  k1 : Inport  Port=2
  Constant : Constant  Value=-1
  Divide : Product  Inputs=*/
  MATLAB Function : MATLAB Function  TreatAsAtomicUnit=on
  Product : Product  Inputs=3
  Out1 : Outport
  wires:
  e1/1 -> Product/2, MATLAB Function/1(u)
  Divide/1 -> Out1/1
  Constant/1 -> Product/1
  k1/1 -> Product/3
  MATLAB Function/1(y) -> Divide/2
  Product/1 -> Divide/1

== system chap05/Subsystem16/Subsystem1/Subsystem3/Subsystem2 ==
  e1 : Inport
  switch : Inport  Port=2
  Constant1 : Constant  Value=0.1
  MATLAB Function : MATLAB Function  TreatAsAtomicUnit=on
  Product{,1..3,6} (5 alike) : Product
  Sqrt : Sqrt  SaturateOnIntegerOverflow=on
  Square : Math  Operator=square  SaturateOnIntegerOverflow=on
  Subsystem : Subsystem
      settings: PortSchema="{\"entries\":[{\"content\":{\"sides\":[{\"content\":{\"connectorIds\":[\"In1\"]},\"type\":\"ConnectorPlacement.EquallySpacedRectSide\",\"uuid\":\"12a3f2f0-a297-420d-b26a-5f62088d5514\"},{\"content\":{\"connectorIds\":[\"Out1\"],\"side\":\"RIGHT\"},\"type\":\"ConnectorPlacement.EquallySpacedRectSide\",\"uuid\":\"62e35448-e0a3-4495-a6db-77deef7aa7b4\"},{\"content\":{\"connectorIds\":[\"In2\"],\"side\":\"TOP\"},\"type\":\"ConnectorPlacement.EquallySpacedRectSide\",\"uuid\":\"3e6c604a-b26b-4ac2-9bdc-2cdec7247e53\"}]},\"type\":\"ConnectorPlacement.EquallySpacedConnector\",\"uuid\":\"6331fe4a-63c7-4003-9b0d-be968a8635fa\"}],\"packageUris\":[\"http://schema.mathworks.com/mf0/Connector/R2020b\"],\"version\":\"1.0\"}"
  Subtract2 : Sum  Inputs=+-
  c1 : Constant  Value=0.1
  c2 : Constant  Value=0.1
  c3 : Constant  Value=0.3
  c4 : Constant  Value=0.3
  k1 : Outport
  k2 : Outport  Port=2
  k3 : Outport  Port=3
  k4 : Outport  Port=4
  wires:
  c2/1 -> Product/2
  Product/1 -> k2/1
  c3/1 -> Product1/1
  Product1/1 -> k3/1
  c4/1 -> Product2/1
  Product2/1 -> k4/1
  c1/1 -> Product3/2
  Product3/1 -> k1/1
  Sqrt/1 -> Product3/1
  Square/1 -> Product2/2
  e1/1 -> MATLAB Function/1(u)
  Product6/1 -> Subtract2/2
  MATLAB Function/1(y) -> Subtract2/1
  Subtract2/1 -> Subsystem/1(In1)
  Constant1/1 -> Product6/1
  switch/1 -> Subsystem/2(switch)
  Subsystem/1(Out1) -> Product6/2, Sqrt/1, Product1/2, Square/1, Product/1

== system chap05/Subsystem16/Subsystem1/Subsystem3/Subsystem3 ==
  e1 : Inport
  k2 : Inport  Port=2
  Constant2 : Constant  Value=-1
  Product2 : Product  Inputs=3
  Out1 : Outport
  wires:
  Product2/1 -> Out1/1
  e1/1 -> Product2/2
  k2/1 -> Product2/3
  Constant2/1 -> Product2/1

== system chap05/Subsystem16/Subsystem1/Subsystem5/Subsystem ==
  switch : Inport
  zt3 : Inport  Port=2
  Constant4 : Constant  Value=0
  Discrete-Time Integrator : DiscreteIntegrator  SampleTime=-1  UpperSaturationLimit=100  LowerSaturationLimit=-100  ICPrevOutput=DiscIntNeverNeededParam  ICPrevScaledInput=DiscIntNeverNeededParam
  Logical Operator : Logic  AllPortsSameDT=off  OutDataTypeStr=boolean
  MATLAB Function : MATLAB Function  TreatAsAtomicUnit=on
  Relational Operator : RelationalOperator  Operator===  OutDataTypeStr=boolean  RndMeth=Simplest
  Saturation1 : Saturate  UpperLimit=0.25  LowerLimit=-0.25
  Sign : Signum
  Sign1 : Signum
  Subsystem : Subsystem
      settings: PortSchema="{\"entries\":[{\"content\":{\"sides\":[{\"content\":{\"connectorIds\":[\"In1\"]},\"type\":\"ConnectorPlacement.EquallySpacedRectSide\",\"uuid\":\"50b1559e-7173-4ba8-93e6-314f6d9df527\"},{\"content\":{\"connectorIds\":[\"Out1\"],\"side\":\"RIGHT\"},\"type\":\"ConnectorPlacement.EquallySpacedRectSide\",\"uuid\":\"be527bac-0bcc-4faf-a185-0382edae0189\"},{\"content\":{\"connectorIds\":[\"In2\"],\"side\":\"TOP\"},\"type\":\"ConnectorPlacement.EquallySpacedRectSide\",\"uuid\":\"4c8ef68d-7cf5-4d15-9758-89dbc1169805\"}]},\"type\":\"ConnectorPlacement.EquallySpacedConnector\",\"uuid\":\"3c2ee67b-c3c9-431a-8107-6d5cd22b236e\"}],\"packageUris\":[\"http://schema.mathworks.com/mf0/Connector/R2020b\"],\"version\":\"1.0\"}"
  Switch : Switch  Criteria=u2 > Threshold
  Out1 : Outport
  wires:
  MATLAB Function/1(y) -> Logical Operator/1
  Relational Operator/1 -> Logical Operator/2
  Constant4/1 -> Switch/1
  Sign1/1 -> Relational Operator/1
  Subsystem/1(Out1) -> Sign1/1, Switch/3
  Saturation1/1 -> Out1/1, MATLAB Function/2(u2)
  Discrete-Time Integrator/1 -> Saturation1/1, MATLAB Function/1(u1), Sign/1
  Sign/1 -> Relational Operator/2
  Logical Operator/1 -> Switch/2
  Switch/1 -> Discrete-Time Integrator/1
  zt3/1 -> Subsystem/1(zt3)
  switch/1 -> Subsystem/2(switch)

== system chap05/Subsystem16/Subsystem1/Subsystem8/Subsystem ==
  In1 : Inport
  switch : Inport  Port=2
  Constant4 : Constant  Value=0
  Switch1 : Switch  Criteria=u2 > Threshold
  Out1 : Outport
  wires:
  In1/1 -> Switch1/1
  Switch1/1 -> Out1/1
  switch/1 -> Switch1/2
  Constant4/1 -> Switch1/3

== system chap05/Subsystem16/Subsystem1/Subsystem8/Subsystem1 ==
  In1 : Inport
  switch : Inport  Port=2
  Constant4 : Constant  Value=0
  Switch1 : Switch  Criteria=u2 > Threshold
  Out1 : Outport
  wires:
  Constant4/1 -> Switch1/3
  switch/1 -> Switch1/2
  Switch1/1 -> Out1/1
  In1/1 -> Switch1/1

== system chap05/Subsystem16/Subsystem1/Subsystem8/Subsystem2 ==
  In1 : Inport
  switch : Inport  Port=2
  Constant4 : Constant  Value=0
  Switch1 : Switch  Criteria=u2 > Threshold
  Out1 : Outport
  wires:
  In1/1 -> Switch1/1
  Switch1/1 -> Out1/1
  switch/1 -> Switch1/2
  Constant4/1 -> Switch1/3

== system chap05/Subsystem16/Subsystem1/Subsystem9/Subsystem ==
  switch : Inport
  zt3 : Inport  Port=2
  Constant4 : Constant  Value=0
  Discrete-Time Integrator : DiscreteIntegrator  SampleTime=-1  UpperSaturationLimit=100  LowerSaturationLimit=-100  ICPrevOutput=DiscIntNeverNeededParam  ICPrevScaledInput=DiscIntNeverNeededParam
  Logical Operator : Logic  AllPortsSameDT=off  OutDataTypeStr=boolean
  MATLAB Function : MATLAB Function  TreatAsAtomicUnit=on
  Relational Operator : RelationalOperator  Operator===  OutDataTypeStr=boolean  RndMeth=Simplest
  Saturation1 : Saturate  UpperLimit=0.25  LowerLimit=-0.25
  Sign : Signum
  Sign1 : Signum
  Subsystem : Subsystem
      settings: PortSchema="{\"entries\":[{\"content\":{\"sides\":[{\"content\":{\"connectorIds\":[\"In1\"]},\"type\":\"ConnectorPlacement.EquallySpacedRectSide\",\"uuid\":\"50b1559e-7173-4ba8-93e6-314f6d9df527\"},{\"content\":{\"connectorIds\":[\"Out1\"],\"side\":\"RIGHT\"},\"type\":\"ConnectorPlacement.EquallySpacedRectSide\",\"uuid\":\"be527bac-0bcc-4faf-a185-0382edae0189\"},{\"content\":{\"connectorIds\":[\"In2\"],\"side\":\"TOP\"},\"type\":\"ConnectorPlacement.EquallySpacedRectSide\",\"uuid\":\"4c8ef68d-7cf5-4d15-9758-89dbc1169805\"}]},\"type\":\"ConnectorPlacement.EquallySpacedConnector\",\"uuid\":\"3c2ee67b-c3c9-431a-8107-6d5cd22b236e\"}],\"packageUris\":[\"http://schema.mathworks.com/mf0/Connector/R2020b\"],\"version\":\"1.0\"}"
  Switch : Switch  Criteria=u2 > Threshold
  Out1 : Outport
  wires:
  zt3/1 -> Subsystem/1(zt3)
  switch/1 -> Subsystem/2(switch)
  Switch/1 -> Discrete-Time Integrator/1
  Logical Operator/1 -> Switch/2
  Sign/1 -> Relational Operator/2
  Discrete-Time Integrator/1 -> Saturation1/1, Sign/1, MATLAB Function/1(u1)
  Saturation1/1 -> MATLAB Function/2(u2), Out1/1
  Subsystem/1(Out1) -> Switch/3, Sign1/1
  Sign1/1 -> Relational Operator/1
  Constant4/1 -> Switch/1
  Relational Operator/1 -> Logical Operator/2
  MATLAB Function/1(y) -> Logical Operator/1

== system chap05/Subsystem16/Subsystem2/Subsystem11/Subsystem ==
  switch : Inport
  zt3 : Inport  Port=2
  Constant4 : Constant  Value=0
  Discrete-Time Integrator : DiscreteIntegrator  SampleTime=-1  UpperSaturationLimit=100  LowerSaturationLimit=-100  ICPrevOutput=DiscIntNeverNeededParam  ICPrevScaledInput=DiscIntNeverNeededParam
  Logical Operator : Logic  AllPortsSameDT=off  OutDataTypeStr=boolean
  MATLAB Function : MATLAB Function  TreatAsAtomicUnit=on
  Relational Operator : RelationalOperator  Operator===  OutDataTypeStr=boolean  RndMeth=Simplest
  Saturation1 : Saturate  UpperLimit=0.25  LowerLimit=-0.25
  Sign : Signum
  Sign1 : Signum
  Subsystem : Subsystem
      settings: PortSchema="{\"entries\":[{\"content\":{\"sides\":[{\"content\":{\"connectorIds\":[\"In1\"]},\"type\":\"ConnectorPlacement.EquallySpacedRectSide\",\"uuid\":\"50b1559e-7173-4ba8-93e6-314f6d9df527\"},{\"content\":{\"connectorIds\":[\"Out1\"],\"side\":\"RIGHT\"},\"type\":\"ConnectorPlacement.EquallySpacedRectSide\",\"uuid\":\"be527bac-0bcc-4faf-a185-0382edae0189\"},{\"content\":{\"connectorIds\":[\"In2\"],\"side\":\"TOP\"},\"type\":\"ConnectorPlacement.EquallySpacedRectSide\",\"uuid\":\"4c8ef68d-7cf5-4d15-9758-89dbc1169805\"}]},\"type\":\"ConnectorPlacement.EquallySpacedConnector\",\"uuid\":\"3c2ee67b-c3c9-431a-8107-6d5cd22b236e\"}],\"packageUris\":[\"http://schema.mathworks.com/mf0/Connector/R2020b\"],\"version\":\"1.0\"}"
  Switch : Switch  Criteria=u2 > Threshold
  Out1 : Outport
  wires:
  MATLAB Function/1(y) -> Logical Operator/1
  Relational Operator/1 -> Logical Operator/2
  Constant4/1 -> Switch/1
  Sign1/1 -> Relational Operator/1
  Subsystem/1(Out1) -> Sign1/1, Switch/3
  Saturation1/1 -> Out1/1, MATLAB Function/2(u2)
  Discrete-Time Integrator/1 -> Saturation1/1, MATLAB Function/1(u1), Sign/1
  Sign/1 -> Relational Operator/2
  Logical Operator/1 -> Switch/2
  Switch/1 -> Discrete-Time Integrator/1
  zt3/1 -> Subsystem/1(zt3)
  switch/1 -> Subsystem/2(switch)

== system chap05/Subsystem16/Subsystem2/Subsystem3/Subsystem ==
  e1 : Inport
  k3 : Inport  Port=2
  k4 : Inport  Port=3
  Add : Sum
  Constant3 : Constant  Value=-1
  Constant4 : Constant  Value=-1
  Discrete-Time Integrator1 : DiscreteIntegrator  SampleTime=-1  ICPrevOutput=DiscIntNeverNeededParam  ICPrevScaledInput=DiscIntNeverNeededParam
  Divide : Product  Inputs=*/
  MATLAB Function : MATLAB Function  TreatAsAtomicUnit=on
  Product3 : Product  Inputs=3
  Product5 : Product  Inputs=3
  z2 : Outport
  wires:
  Constant4/1 -> Product5/1
  Product5/1 -> Add/2
  Discrete-Time Integrator1/1 -> z2/1
  k3/1 -> Product3/3
  k4/1 -> Product5/3
  Divide/1 -> Add/1
  Add/1 -> Discrete-Time Integrator1/1
  Constant3/1 -> Product3/1
  e1/1 -> Product5/2, MATLAB Function/1(u), Product3/2
  MATLAB Function/1(y) -> Divide/2
  Product3/1 -> Divide/1

== system chap05/Subsystem16/Subsystem2/Subsystem3/Subsystem1 ==
  e1 : Inport
  k1 : Inport  Port=2
  Constant : Constant  Value=-1
  Divide : Product  Inputs=*/
  MATLAB Function : MATLAB Function  TreatAsAtomicUnit=on
  Product : Product  Inputs=3
  Out1 : Outport
  wires:
  e1/1 -> Product/2, MATLAB Function/1(u)
  Divide/1 -> Out1/1
  Constant/1 -> Product/1
  k1/1 -> Product/3
  MATLAB Function/1(y) -> Divide/2
  Product/1 -> Divide/1

== system chap05/Subsystem16/Subsystem2/Subsystem3/Subsystem2 ==
  e1 : Inport
  switch : Inport  Port=2
  Constant1 : Constant  Value=0.1
  MATLAB Function : MATLAB Function  TreatAsAtomicUnit=on
  Product{,1..3,6} (5 alike) : Product
  Sqrt : Sqrt  SaturateOnIntegerOverflow=on
  Square : Math  Operator=square  SaturateOnIntegerOverflow=on
  Subsystem : Subsystem
      settings: PortSchema="{\"entries\":[{\"content\":{\"sides\":[{\"content\":{\"connectorIds\":[\"In1\"]},\"type\":\"ConnectorPlacement.EquallySpacedRectSide\",\"uuid\":\"12a3f2f0-a297-420d-b26a-5f62088d5514\"},{\"content\":{\"connectorIds\":[\"Out1\"],\"side\":\"RIGHT\"},\"type\":\"ConnectorPlacement.EquallySpacedRectSide\",\"uuid\":\"62e35448-e0a3-4495-a6db-77deef7aa7b4\"},{\"content\":{\"connectorIds\":[\"In2\"],\"side\":\"TOP\"},\"type\":\"ConnectorPlacement.EquallySpacedRectSide\",\"uuid\":\"3e6c604a-b26b-4ac2-9bdc-2cdec7247e53\"}]},\"type\":\"ConnectorPlacement.EquallySpacedConnector\",\"uuid\":\"6331fe4a-63c7-4003-9b0d-be968a8635fa\"}],\"packageUris\":[\"http://schema.mathworks.com/mf0/Connector/R2020b\"],\"version\":\"1.0\"}"
  Subtract2 : Sum  Inputs=+-
  c1 : Constant  Value=0.1
  c2 : Constant  Value=0.1
  c3 : Constant  Value=0.3
  c4 : Constant  Value=0.3
  k1 : Outport
  k2 : Outport  Port=2
  k3 : Outport  Port=3
  k4 : Outport  Port=4
  wires:
  c2/1 -> Product/2
  Product/1 -> k2/1
  c3/1 -> Product1/1
  Product1/1 -> k3/1
  c4/1 -> Product2/1
  Product2/1 -> k4/1
  c1/1 -> Product3/2
  Product3/1 -> k1/1
  Sqrt/1 -> Product3/1
  Square/1 -> Product2/2
  e1/1 -> MATLAB Function/1(u)
  Product6/1 -> Subtract2/2
  MATLAB Function/1(y) -> Subtract2/1
  Subtract2/1 -> Subsystem/1(In1)
  Constant1/1 -> Product6/1
  switch/1 -> Subsystem/2(switch)
  Subsystem/1(Out1) -> Product6/2, Sqrt/1, Product1/2, Square/1, Product/1

== system chap05/Subsystem16/Subsystem2/Subsystem3/Subsystem3 ==
  e1 : Inport
  k2 : Inport  Port=2
  Constant2 : Constant  Value=-1
  Product2 : Product  Inputs=3
  Out1 : Outport
  wires:
  Product2/1 -> Out1/1
  e1/1 -> Product2/2
  k2/1 -> Product2/3
  Constant2/1 -> Product2/1

== system chap05/Subsystem16/Subsystem2/Subsystem4/Subsystem ==
  switch : Inport
  zt3 : Inport  Port=2
  Constant4 : Constant  Value=0
  Discrete-Time Integrator : DiscreteIntegrator  SampleTime=-1  UpperSaturationLimit=100  LowerSaturationLimit=-100  ICPrevOutput=DiscIntNeverNeededParam  ICPrevScaledInput=DiscIntNeverNeededParam
  Logical Operator : Logic  AllPortsSameDT=off  OutDataTypeStr=boolean
  MATLAB Function : MATLAB Function  TreatAsAtomicUnit=on
  Relational Operator : RelationalOperator  Operator===  OutDataTypeStr=boolean  RndMeth=Simplest
  Saturation1 : Saturate  UpperLimit=0.25  LowerLimit=-0.25
  Sign : Signum
  Sign1 : Signum
  Subsystem : Subsystem
      settings: PortSchema="{\"entries\":[{\"content\":{\"sides\":[{\"content\":{\"connectorIds\":[\"In1\"]},\"type\":\"ConnectorPlacement.EquallySpacedRectSide\",\"uuid\":\"50b1559e-7173-4ba8-93e6-314f6d9df527\"},{\"content\":{\"connectorIds\":[\"Out1\"],\"side\":\"RIGHT\"},\"type\":\"ConnectorPlacement.EquallySpacedRectSide\",\"uuid\":\"be527bac-0bcc-4faf-a185-0382edae0189\"},{\"content\":{\"connectorIds\":[\"In2\"],\"side\":\"TOP\"},\"type\":\"ConnectorPlacement.EquallySpacedRectSide\",\"uuid\":\"4c8ef68d-7cf5-4d15-9758-89dbc1169805\"}]},\"type\":\"ConnectorPlacement.EquallySpacedConnector\",\"uuid\":\"3c2ee67b-c3c9-431a-8107-6d5cd22b236e\"}],\"packageUris\":[\"http://schema.mathworks.com/mf0/Connector/R2020b\"],\"version\":\"1.0\"}"
  Switch : Switch  Criteria=u2 > Threshold
  Out1 : Outport
  wires:
  MATLAB Function/1(y) -> Logical Operator/1
  Relational Operator/1 -> Logical Operator/2
  Constant4/1 -> Switch/1
  Sign1/1 -> Relational Operator/1
  Subsystem/1(Out1) -> Sign1/1, Switch/3
  Saturation1/1 -> Out1/1, MATLAB Function/2(u2)
  Discrete-Time Integrator/1 -> Saturation1/1, MATLAB Function/1(u1), Sign/1
  Sign/1 -> Relational Operator/2
  Logical Operator/1 -> Switch/2
  Switch/1 -> Discrete-Time Integrator/1
  zt3/1 -> Subsystem/1(zt3)
  switch/1 -> Subsystem/2(switch)

== system chap05/Subsystem16/Subsystem2/Subsystem8/Subsystem ==
  In1 : Inport
  switch : Inport  Port=2
  Constant4 : Constant  Value=0
  Switch1 : Switch  Criteria=u2 > Threshold
  Out1 : Outport
  wires:
  In1/1 -> Switch1/1
  Switch1/1 -> Out1/1
  switch/1 -> Switch1/2
  Constant4/1 -> Switch1/3

== system chap05/Subsystem16/Subsystem2/Subsystem8/Subsystem1 ==
  In1 : Inport
  switch : Inport  Port=2
  Constant4 : Constant  Value=0
  Switch1 : Switch  Criteria=u2 > Threshold
  Out1 : Outport
  wires:
  Constant4/1 -> Switch1/3
  switch/1 -> Switch1/2
  Switch1/1 -> Out1/1
  In1/1 -> Switch1/1

== system chap05/Subsystem16/Subsystem2/Subsystem8/Subsystem2 ==
  In1 : Inport
  switch : Inport  Port=2
  Constant4 : Constant  Value=0
  Switch1 : Switch  Criteria=u2 > Threshold
  Out1 : Outport
  wires:
  In1/1 -> Switch1/1
  Switch1/1 -> Out1/1
  switch/1 -> Switch1/2
  Constant4/1 -> Switch1/3
